simulink model "untitled"  (R2020b)
settings: Solver=FixedStepAuto  StartTime=0.0  StopTime=10.0  FixedStep=0.01  RelTol=1e-3
settings Model: Creator=ricky  LastModifiedBy=ricky

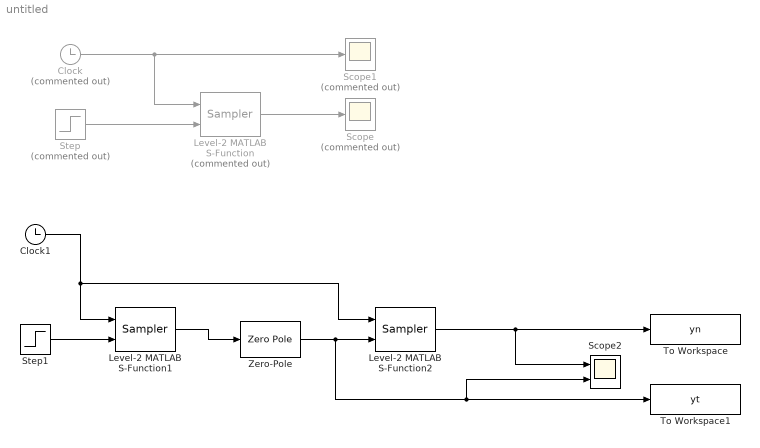
== system untitled ==
  Clock : Clock  Commented=on
  Clock1 : Clock
  Level-2 MATLAB S-Function : M-S-Function  Commented=on  FunctionName=Sampler  Parameters=1,0
  Level-2 MATLAB S-Function1 : M-S-Function  FunctionName=Sampler  Parameters=1,0
  Level-2 MATLAB S-Function2 : M-S-Function  FunctionName=Sampler  Parameters=1,0
  Scope : Scope  Commented=on
  Scope1 : Scope  Commented=on
  Scope2 : Scope  NumInputPorts=2
  Step : Step  Commented=on  SampleTime=0
  Step1 : Step  Time=0  SampleTime=0
  To Workspace : ToWorkspace  VariableName=yn  SaveFormat=Timeseries  SampleTime=-1
  To Workspace1 : ToWorkspace  VariableName=yt  SaveFormat=Timeseries  SampleTime=-1
  Zero-Pole : ZeroPole  Zeros=[]  Poles=[-1]
  wires:
  Clock/1 -> Scope1/1, Level-2 MATLAB S-Function/1
  Level-2 MATLAB S-Function/1 -> Scope/1
  Step/1 -> Level-2 MATLAB S-Function/2
  Level-2 MATLAB S-Function2/1 -> Scope2/1, To Workspace/1
  Zero-Pole/1 -> Level-2 MATLAB S-Function2/2, Scope2/2, To Workspace1/1
  Clock1/1 -> Level-2 MATLAB S-Function2/1, Level-2 MATLAB S-Function1/1
  Level-2 MATLAB S-Function1/1 -> Zero-Pole/1
  Step1/1 -> Level-2 MATLAB S-Function1/2
